simulink library "mad_lib_template"  (R2026a)
settings: Solver=VariableStepAuto
values from neighbouring files (symbols this model uses):
  P_dt = 25e-3    (= 0.025)    [s06_data.m]
undefined symbols (not defined in the file or in its folder): P_e_P0, P_e_param, P_e_Qu, P_e_R, P_e_x0
settings Model: Creator=ftraenkle  LastModifiedBy=thele

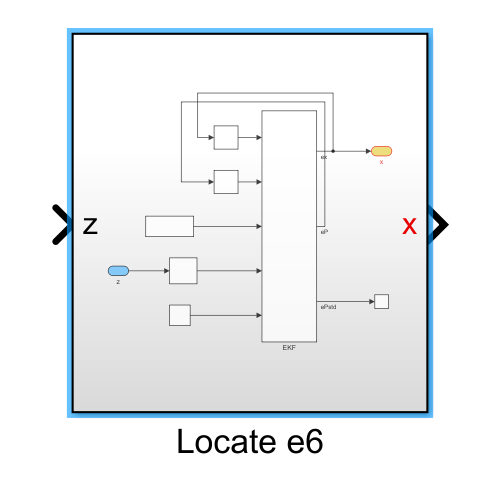
[thumbnail: Simulink's stored preview of the top-level diagram]
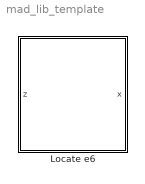
== system mad_lib_template ==
  Locate e6 : Subsystem  SystemSampleTime=P_dt

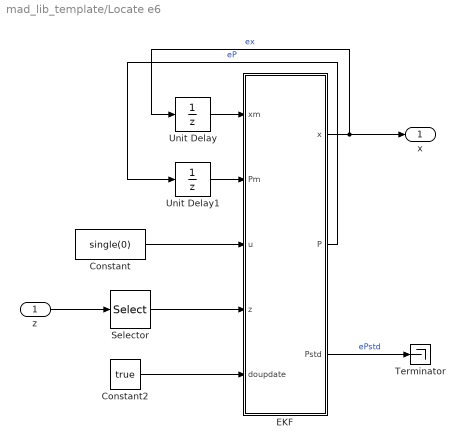
== system mad_lib_template/Locate e6 ==
  z : Inport
  Constant : Constant  Value=single(0)
  Constant2 : Constant  Value=true
  EKF : MATLAB Function  TreatAsAtomicUnit=on
  Selector : Selector  InputPortWidth=3  IndexOptions=Index vector (dialog)  Indices=[1 2]  OutputSizes=1
  Terminator : Terminator
  Unit Delay : UnitDelay  InitialCondition=P_e_x0  SampleTime=-1
  Unit Delay1 : UnitDelay  InitialCondition=P_e_P0  SampleTime=-1
  x : Outport
  wires:
  Constant/1 -> EKF/3(u)
  Selector/1 -> EKF/4(z)
  EKF/2(P) -> Unit Delay1/1  "eP"
  EKF/1(x) -> x/1, Unit Delay/1  "ex"
  z/1 -> Selector/1
  Unit Delay1/1 -> EKF/2(Pm)
  EKF/3(Pstd) -> Terminator/1  "ePstd"
  Unit Delay/1 -> EKF/1(xm)
  Constant2/1 -> EKF/5(doupdate)

== matlab function mad_lib_template/Locate e6/EKF ==
  data: xm input single; Pm input single; u input; x output; z input; doupdate input; P output; P_e_Qu parameter; P_e_R parameter; P_e_param parameter; Pstd output
function [ x , P , Pstd ] = ekf(xm, Pm, u, z, doupdate, ...
    P_e_Qu, P_e_R, P_e_param) 

n = length(xm);

x = e6_nonlinsys_f(xm, u, P_e_param);
y = e6_nonlinsys_h(x, u, P_e_param);
[ A, B, C, G ] = e6_linsys(x, xm, u, P_e_param);
P = A * Pm * A' + G * P_e_Qu * G';

if doupdate
    P12 = P * C';
    K = P12 / (C * P12 + P_e_R); % Kalman filter gain
    e = z - y;
    x = x + K * e; % state estimate
    T = eye(n, 'single') - K * C;
    P = T * P * T' + K * P_e_R * K'; % Joseph form   
end
Pstd = sqrt(diag(P) .* diag(P));
end
